simulink model "VOR_hold"  (R2023b)
settings: Solver=VariableStepAuto  StartTime=0.0  StopTime=10.0  RelTol=1e-3
undefined symbols (not defined in the file or in its folder): K_p, K_phi, K_psi, K_r, trim_control_lo, trim_state_lin, trim_state_lo, VOR_sys
libraries: slpidlib x2
settings Model: Creator=Albertlakers  LastModifiedBy=Albertlakers

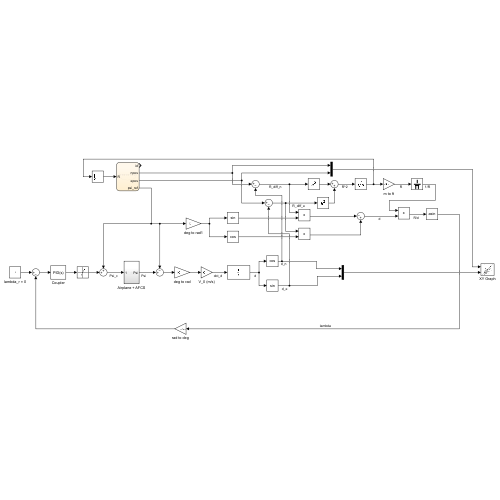
[thumbnail: Simulink's stored preview of the top-level diagram]
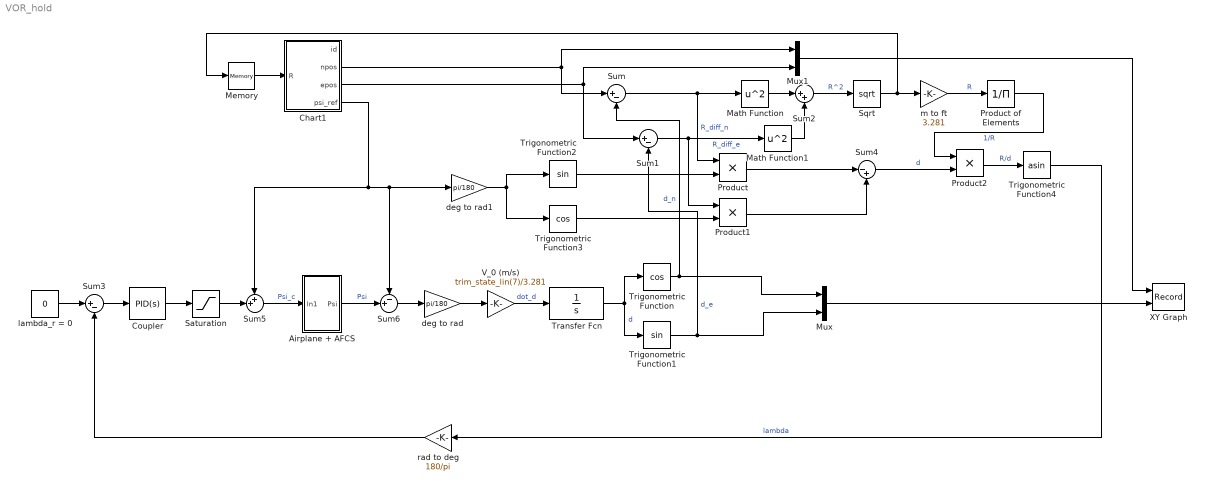
== system VOR_hold ==
  Airplane + AFCS : Subsystem
  Chart1 : Stateflow chart  TreatAsAtomicUnit=on
  Coupler : slpidlib/PID Controller  Controller=PID  Form=Parallel  TimeDomain=Continuous-time  UseExternalTs=off  SampleTime=-1  IntegratorMethod=Forward Euler  FilterMethod=Forward Euler  ControllerParametersSource=internal  P=1  I=1  UseKiTs=off  D=0  N=100  UseFilter=on  TunerSelectOption=Transfer Function Based (PID Tuner App)  InitialConditionSource=internal  InitialConditionForIntegrator=0  InitialConditionForFilter=0  DifferentiatorICPrevScaledInput=0  ExternalReset=none  TrackingMode=off  Kt=1  LimitOutput=off  SatLimitsSource=internal  UpperSaturationLimit=inf  LowerSaturationLimit=-inf  LinearizeAsGain=on  AntiWindupMode=none  Kb=1  LimitIntegrator=off  UpperIntegratorSaturationLimit=inf  LowerIntegratorSaturationLimit=-inf  POutMin=[]  POutMax=[]  IOutMin=[]  IOutMax=[]  DOutMin=[]  DOutMax=[]  NOutMin=[]  NOutMax=[]  SumOutMin=[]  SumOutMax=[]  SaturationOutMin=[]  SaturationOutMax=[]  PParamMin=[]  PParamMax=[]  IParamMin=[]  IParamMax=[]  DParamMin=[]  DParamMax=[]  NParamMin=[]  NParamMax=[]  KbParamMin=[]  KbParamMax=[]  KtParamMin=[]  KtParamMax=[]  KbOutMin=[]  KbOutMax=[]  KtOutMin=[]  KtOutMax=[]  IntegratorOutMin=[]  IntegratorOutMax=[]  FilterOutMin=[]  FilterOutMax=[]  SumI1OutMin=[]  SumI1OutMax=[]  SumI2OutMin=[]  SumI2OutMax=[]  SumI3OutMin=[]  SumI3OutMax=[]  SumI4OutMin=[]  SumI4OutMax=[]  SumDOutMin=[]  SumDOutMax=[]  DifferentiatorOutMin=[]  DifferentiatorOutMax=[]  FilterDiffOutCoefMin=[]  FilterDiffOutCoefMax=[]  ReciprocalOutMin=[]  ReciprocalOutMax=[]  SumDenOutMin=[]  SumDenOutMax=[]  SumNumOutMin=[]  SumNumOutMax=[]  DivideOutMin=[]  DivideOutMax=[]  UdiffTsProdOutMin=[]  UdiffTsProdOutMax=[]  NTsProdOutMin=[]  NTsProdOutMax=[]  UintegralTsProdOutMin=[]  UintegralTsProdOutMax=[]  UngainTsProdOutMin=[]  UngainTsProdOutMax=[]  ClampingZeroOutDataTypeStr=Inherit: Inherit via back propagation  ClampingZeroOutMin=[]  ClampingZeroOutMax=[]  FilterDenConstantOutDataTypeStr=Inherit: Inherit via back propagation  FilterDenConstantOutMin=[]  FilterDenConstantOutMax=[]  PCopyOutDataTypeStr=Inherit: Inherit via back propagation  PCopyOutMin=[]  PCopyOutMax=[]  NCopyOutDataTypeStr=Inherit: Inherit via back propagation  NCopyOutMin=[]  NCopyOutMax=[]  IntegratorContinuousStateAttributes=''  IntegratorStateMustResolveToSignalObject=off  IntegratorRTWStateStorageClass=Auto  FilterContinuousStateAttributes=''  FilterStateMustResolveToSignalObject=off  FilterRTWStateStorageClass=Auto  ParallelPVariant=InternalParameters  IdealPVariant=Disabled  IVariant=InternalParameters  DVariant=InternalParameters  IntegratorVariant=Continuous  SatVariant=Disabled  AWVariant=Passthrough  PCopyVariant=Disabled  TRVariant=Disabled  FdbkBlocksVariant=Forward  IdealPFdbkVariant=Disabled  SatFdbkVariant=Disabled  DerivativeFilterVariant=ContFilter  NVariant=InternalParameters  NCopyVariant=Disabled  FilterICVariant=InternalICsFilter  IntegratorICVariant=InternalICs  ExternalResetVariant=Disabled  TRSumVariant=Passthrough  SumFdbkVariant=Disabled  SumVariant=Sum_PID  TsampFilterVariant=InternalTs  TsampNgainVariant=Passthrough  TsampIntegralVariant=Disabled_SignalSpec  ExternalSaturationOutDataTypeStr=Inherit: Same as second input
  Math Function : Math  Operator=square
  Math Function1 : Math  Operator=square
  Memory : Memory
  Mux : Mux  Inputs=2
  Mux1 : Mux  Inputs=2
  Product : Product
  Product of Elements : Product  Inputs=/
  Product1 : Product
  Product2 : Product
  Saturation : Saturate  UpperLimit=90  LowerLimit=-90
  Sqrt : Sqrt
  Sum : Sum  Inputs=|+-
  Sum1 : Sum  Inputs=|+-
  Sum2 : Sum  Inputs=|++
  Sum3 : Sum  Inputs=|+-
  Sum4 : Sum  Inputs=|-+
  Sum5 : Sum  Inputs=++|
  Sum6 : Sum  Inputs=-+|
  Transfer Fcn : TransferFcn  Denominator=[1 0]
  Trigonometric Function : Trigonometry  Operator=cos
  Trigonometric Function1 : Trigonometry
  Trigonometric Function2 : Trigonometry
  Trigonometric Function3 : Trigonometry  Operator=cos
  Trigonometric Function4 : Trigonometry  Operator=asin
  V_0 (m/s) : Gain  Gain=trim_state_lin(7)/3.281
  XY Graph : Record  FileSettingsInternal="{\"entries\":[{\"content\":{\"excelSettings\":{\"content\":{},\"type\":\"Streamout.ExcelSettings\"}},\"type\":\"Streamout.FileSettingStorage\",\"uuid\":\"\"}],\"packageUris\":[\"http:\\/\\/schema.mathworks.com\\/mf0\\/streamout_blocks\\/R2020a\"],\"version\":\"1.0\"}"  Layout=[1 1]  SignalsInternal="{\"entries\":[{\"content\":{\"signals\":[{\"content\":{\"blockPath\":[],\"dimensions\":[1],\"domain\":\"\",\"lineColor\":\"#a2142f\",\"plots\":[1],\"port\":1,\"signalID\":17,\"signalName\":\"XY Graph:1\"},\"type\":\"RecordBlkView.Signal\",\"uuid\":\"\"},{\"content\":{\"blockPath\":[],\"dimensions\":[1],\"domain\":\"\",\"lineColor\":\"#139fff\",\"plots\":[1],\"port\":2,\"signalID\":20,\"signalName\":\"XY Graph:2\"},\"type\":\"RecordBlkView.Signal\",\"uuid\":\"\"}]},\"type\":\"RecordBlkView.InputSignals\",\"uuid\":\"\"}],\"packageUris\":[\"http:\\/\\/schema.mathworks.com\\/mf0\\/streamout_blocks\\/R2020a\"],\"version\":\"1.0\"}"  VisualizationBindings="{\"xyplotplugin\":{\"info\":[{\"series\":[{\"bindingParametersList\":[{\"parameter\":\"X-Axis\",\"signalID\":17,\"signalName\":\"XY Graph:1\"},{\"parameter\":\"Y-Axis\",\"signalID\":20,\"signalName\":\"XY Graph:2\"}],\"seriesID\":64857}],\"subplotID\":1}]}}"  CompatibilityTag=XY
  deg to rad : Gain  Gain=pi/180
  deg to rad1 : Gain  Gain=pi/180
  lambda_r = 0 : Constant  Value=0
  m to ft : Gain  Gain=3.281
  rad to deg : Gain  Gain=180/pi
  wires:
  Chart1/3(epos) -> Sum1/1, Mux1/2
  Memory/1 -> Chart1/1(R)
  Chart1/4(psi_ref) -> deg to rad1/1, Sum6/1, Sum5/1
  Chart1/2(npos) -> Sum/1, Mux1/1
  Sqrt/1 -> m to ft/1, Memory/1
  V_0 (m/s)/1 -> Transfer Fcn/1  "dot_d"
  deg to rad/1 -> V_0 (m/s)/1
  Transfer Fcn/1 -> Trigonometric Function1/1, Trigonometric Function/1  "d"
  Trigonometric Function/1 -> Mux/1, Sum/2  "d_n"
  Trigonometric Function1/1 -> Mux/2, Sum1/2  "d_e"
  Mux/1 -> XY Graph/2
  Mux1/1 -> XY Graph/1
  Sum/1 -> Product/1, Math Function/1  "R_diff_n"
  Sum1/1 -> Math Function1/1, Product1/1  "R_diff_e"
  Sum2/1 -> Sqrt/1  "R^2"
  Math Function/1 -> Sum2/1
  Math Function1/1 -> Sum2/2
  m to ft/1 -> Product of Elements/1  "R"
  Sum3/1 -> Coupler/1
  Coupler/1 -> Saturation/1
  lambda_r = 0/1 -> Sum3/1
  deg to rad1/1 -> Trigonometric Function2/1, Trigonometric Function3/1
  Trigonometric Function2/1 -> Product/2
  Trigonometric Function3/1 -> Product1/2
  Product/1 -> Sum4/1
  Product1/1 -> Sum4/2
  Product of Elements/1 -> Product2/1  "1/R"
  Sum4/1 -> Product2/2  "d"
  Product2/1 -> Trigonometric Function4/1  "R/d"
  Trigonometric Function4/1 -> rad to deg/1  "lambda"
  rad to deg/1 -> Sum3/2
  Saturation/1 -> Sum5/2
  Sum5/1 -> Airplane + AFCS/1(In1)  "Psi_c"
  Airplane + AFCS/1(Psi) -> Sum6/2  "Psi"
  Sum6/1 -> deg to rad/1

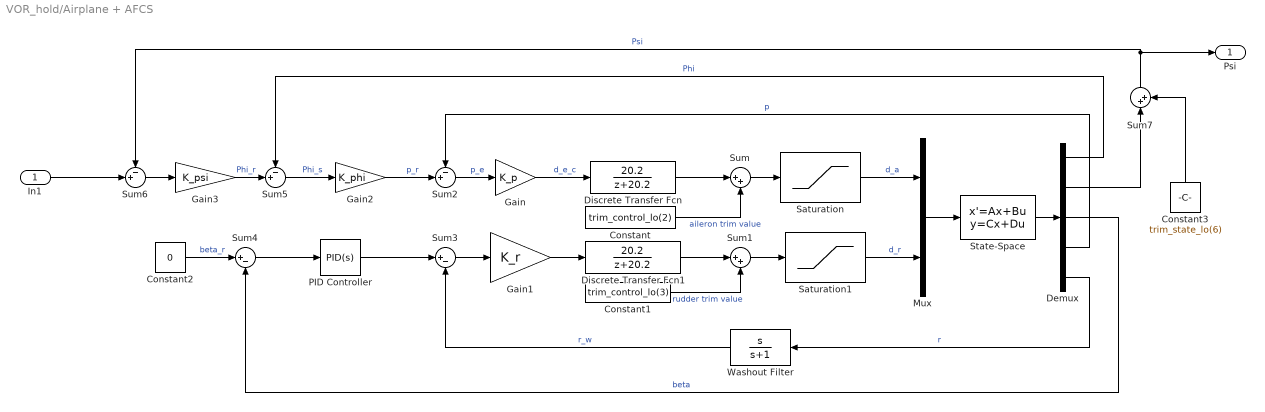
== system VOR_hold/Airplane + AFCS ==
  In1 : Inport
  Constant : Constant  Value=trim_control_lo(2)
  Constant1 : Constant  Value=trim_control_lo(3)
  Constant2 : Constant  Value=0
  Constant3 : Constant  Value=trim_state_lo(6)
  Demux : Demux  Outputs=5
  Discrete Transfer Fcn : DiscreteTransferFcn  Numerator=[20.2]  Denominator=[1 20.2]
  Discrete Transfer Fcn1 : DiscreteTransferFcn  Numerator=[20.2]  Denominator=[1 20.2]
  Gain : Gain  Gain=K_p
  Gain1 : Gain  Gain=K_r
  Gain2 : Gain  Gain=K_phi
  Gain3 : Gain  Gain=K_psi
  Mux : Mux  Inputs=2
  PID Controller : slpidlib/PID Controller  Controller=PID  Form=Parallel  TimeDomain=Continuous-time  UseExternalTs=off  SampleTime=-1  IntegratorMethod=Forward Euler  FilterMethod=Forward Euler  ControllerParametersSource=internal  P=1  I=1  UseKiTs=off  D=0  N=100  UseFilter=on  TunerSelectOption=Transfer Function Based (PID Tuner App)  InitialConditionSource=internal  InitialConditionForIntegrator=0  InitialConditionForFilter=0  DifferentiatorICPrevScaledInput=0  ExternalReset=none  TrackingMode=off  Kt=1  LimitOutput=off  SatLimitsSource=internal  UpperSaturationLimit=inf  LowerSaturationLimit=-inf  LinearizeAsGain=on  AntiWindupMode=none  Kb=1  LimitIntegrator=off  UpperIntegratorSaturationLimit=inf  LowerIntegratorSaturationLimit=-inf  POutMin=[]  POutMax=[]  IOutMin=[]  IOutMax=[]  DOutMin=[]  DOutMax=[]  NOutMin=[]  NOutMax=[]  SumOutMin=[]  SumOutMax=[]  SaturationOutMin=[]  SaturationOutMax=[]  PParamMin=[]  PParamMax=[]  IParamMin=[]  IParamMax=[]  DParamMin=[]  DParamMax=[]  NParamMin=[]  NParamMax=[]  KbParamMin=[]  KbParamMax=[]  KtParamMin=[]  KtParamMax=[]  KbOutMin=[]  KbOutMax=[]  KtOutMin=[]  KtOutMax=[]  IntegratorOutMin=[]  IntegratorOutMax=[]  FilterOutMin=[]  FilterOutMax=[]  SumI1OutMin=[]  SumI1OutMax=[]  SumI2OutMin=[]  SumI2OutMax=[]  SumI3OutMin=[]  SumI3OutMax=[]  SumI4OutMin=[]  SumI4OutMax=[]  SumDOutMin=[]  SumDOutMax=[]  DifferentiatorOutMin=[]  DifferentiatorOutMax=[]  FilterDiffOutCoefMin=[]  FilterDiffOutCoefMax=[]  ReciprocalOutMin=[]  ReciprocalOutMax=[]  SumDenOutMin=[]  SumDenOutMax=[]  SumNumOutMin=[]  SumNumOutMax=[]  DivideOutMin=[]  DivideOutMax=[]  UdiffTsProdOutMin=[]  UdiffTsProdOutMax=[]  NTsProdOutMin=[]  NTsProdOutMax=[]  UintegralTsProdOutMin=[]  UintegralTsProdOutMax=[]  UngainTsProdOutMin=[]  UngainTsProdOutMax=[]  ClampingZeroOutDataTypeStr=Inherit: Inherit via back propagation  ClampingZeroOutMin=[]  ClampingZeroOutMax=[]  FilterDenConstantOutDataTypeStr=Inherit: Inherit via back propagation  FilterDenConstantOutMin=[]  FilterDenConstantOutMax=[]  PCopyOutDataTypeStr=Inherit: Inherit via back propagation  PCopyOutMin=[]  PCopyOutMax=[]  NCopyOutDataTypeStr=Inherit: Inherit via back propagation  NCopyOutMin=[]  NCopyOutMax=[]  IntegratorContinuousStateAttributes=''  IntegratorStateMustResolveToSignalObject=off  IntegratorRTWStateStorageClass=Auto  FilterContinuousStateAttributes=''  FilterStateMustResolveToSignalObject=off  FilterRTWStateStorageClass=Auto  ParallelPVariant=InternalParameters  IdealPVariant=Disabled  IVariant=InternalParameters  DVariant=InternalParameters  IntegratorVariant=Continuous  SatVariant=Disabled  AWVariant=Passthrough  PCopyVariant=Disabled  TRVariant=Disabled  FdbkBlocksVariant=Forward  IdealPFdbkVariant=Disabled  SatFdbkVariant=Disabled  DerivativeFilterVariant=ContFilter  NVariant=InternalParameters  NCopyVariant=Disabled  FilterICVariant=InternalICsFilter  IntegratorICVariant=InternalICs  ExternalResetVariant=Disabled  TRSumVariant=Passthrough  SumFdbkVariant=Disabled  SumVariant=Sum_PID  TsampFilterVariant=InternalTs  TsampNgainVariant=Passthrough  TsampIntegralVariant=Disabled_SignalSpec  ExternalSaturationOutDataTypeStr=Inherit: Same as second input
  Saturation : Saturate  UpperLimit=21.5  LowerLimit=-21.5
  Saturation1 : Saturate  UpperLimit=30  LowerLimit=-30
  State-Space : StateSpace  A=VOR_sys.A  B=VOR_sys.B  C=VOR_sys.C  D=VOR_sys.D  InitialCondition=0  ParameterTunability=Unconstrained  ContinuousStateAttributes='Phi' 'Psi' 'beta' 'p' 'r'
  Sum : Sum  Inputs=|++
  Sum1 : Sum  Inputs=|++
  Sum2 : Sum  Inputs=-+|
  Sum3 : Sum  Inputs=|+-
  Sum4 : Sum  Inputs=|+-
  Sum5 : Sum  Inputs=-+|
  Sum6 : Sum  Inputs=-+|
  Sum7 : Sum  Inputs=|++
  Washout Filter : TransferFcn  Numerator=[1 0]  Denominator=[1 1]
  Psi : Outport
  wires:
  Demux/3 -> Sum4/2  "beta"
  Demux/5 -> Washout Filter/1  "r"
  In1/1 -> Sum6/2
  Discrete Transfer Fcn/1 -> Sum/1
  Sum7/1 -> Psi/1, Sum6/1  "Psi"
  Sum/1 -> Saturation/1
  Sum5/1 -> Gain2/1  "Phi_s"
  Demux/4 -> Sum2/1  "p"
  Constant/1 -> Sum/2  "aileron trim value"
  Constant1/1 -> Sum1/2  "rudder trim value"
  State-Space/1 -> Demux/1
  Discrete Transfer Fcn1/1 -> Sum1/1
  Gain1/1 -> Discrete Transfer Fcn1/1
  Gain2/1 -> Sum2/2  "p_r"
  Washout Filter/1 -> Sum3/2  "r_w"
  Mux/1 -> State-Space/1
  Constant2/1 -> Sum4/1  "beta_r"
  PID Controller/1 -> Sum3/1
  Sum2/1 -> Gain/1  "p_e"
  Saturation/1 -> Mux/1  "d_a"
  Sum6/1 -> Gain3/1
  Sum3/1 -> Gain1/1
  Gain3/1 -> Sum5/2  "Phi_r"
  Demux/1 -> Sum5/1  "Phi"
  Gain/1 -> Discrete Transfer Fcn/1  "d_e_c"
  Saturation1/1 -> Mux/2  "d_r"
  Demux/2 -> Sum7/1
  Constant3/1 -> Sum7/2
  Sum4/1 -> PID Controller/1
  Sum1/1 -> Saturation1/1

== stateflow chart VOR_hold/Chart1 ==
  settings: updateMethod=DISCRETE  sampleTime=0.1
  state beacon1
    id=1;
    npos=15000;
    epos=15000;
    psi_ref=45;
  state beacon2
    id=2;
    npos=0;
    epos=30000;
    psi_ref=135;
  state beacon3
    id=3;
    npos=-15000;
    epos=30000;
    psi_ref=180;
  state beacon4
    id=4;
    npos=-30000;
    epos=45000;
    psi_ref=135;
  state beacon5
    id=5;
    npos=0;
    epos=0;
    psi_ref=0;
  (default) -> beacon1
  beacon2 -> beacon3 : [R<5000]
  beacon3 -> beacon4 : [R<5000]
  beacon1 -> beacon2 : [R<5000]
  beacon4 -> beacon5 : [R<5000]
  beacon5 -> beacon1 : [R<5000]
  data: R input; id output; npos output; epos output; psi_ref output
